simulink model "q4"  (R2024b)
settings: Solver=VariableStepAuto  StartTime=0.0  StopTime=5  RelTol=1e-3
settings Model: Creator=32602  LastModifiedBy=32602

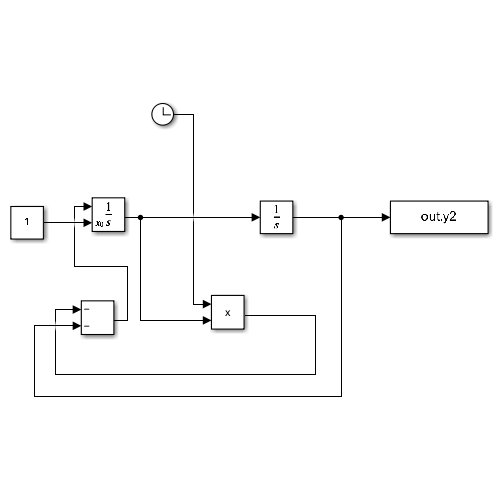
[thumbnail: Simulink's stored preview of the top-level diagram]
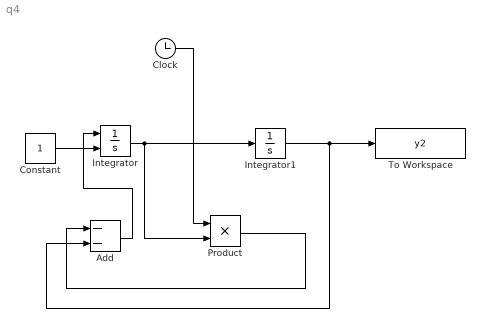
== system q4 ==
  Add : Sum  Inputs=--
  Clock : Clock
  Constant : Constant
  Integrator : Integrator  InitialConditionSource=external
  Integrator1 : Integrator
  Product : Product
  To Workspace : ToWorkspace  VariableName=y2  SaveFormat=Timeseries  SampleTime=0.01
  wires:
  Integrator1/1 -> To Workspace/1, Add/2
  Clock/1 -> Product/1
  Integrator/1 -> Integrator1/1, Product/2
  Product/1 -> Add/1
  Add/1 -> Integrator/1
  Constant/1 -> Integrator/2
